simulink model "dcpController"  (R2016b)
settings: Solver=ode5  StartTime=0.0  StopTime=inf  FixedStep=0.001  RelTol=1e-3  EnableMultiTasking=on
undefined symbols (not defined in the file): robot, Standard_Devices, UDP_Protocol
libraries: dcpctrl x15, simulink x7, kukaslxctrl x1, sldrtlib x1
settings Model: SimulationMode=external  Creator=julianleland  LastModifiedBy=julianleland
settings OptimizationCC: LifeSpan=inf
settings DebuggingCC: SFUnexpectedBacktrackingDiag=warning  SFNoUnconditionalDefaultTransitionDiag=warning  SFExecutionAtInitializationDiag=none
settings HardwareCC: ProdBitPerLong=64  ProdHWDeviceType=Intel->x86-64 (Mac OS X)  TargetBitPerLong=64  TargetBitPerPointer=64  TargetIntDivRoundTo=Zero  TargetEndianess=LittleEndian  TargetWordSize=64  TargetHWDeviceType=Intel->x86-64
settings RTWCC: SystemTargetFile=sldrt.tlc  TemplateMakefile=sldrt.tmf  Description=Simulink Desktop Real-Time  RTWCompilerOptimization=on
settings CodeAppCC: MaxIdLength=95
settings SimulinkDesktopRealTimeCC: TargetPreCompLibLocation=/Applications/MATLAB_R2016b.app/toolbox/sldrt/lib/maci64  TargetLangStandard=C89/C90 (ANSI)  SupportVariableSizeSignals=off
settings ConfigComp: CovMetricSettings=dw  CovHtmlReporting=on  CovSaveCumulativeToWorkspaceVar=on  CovSaveSingleToWorkspaceVar=on  CovExternalEMLEnable=off

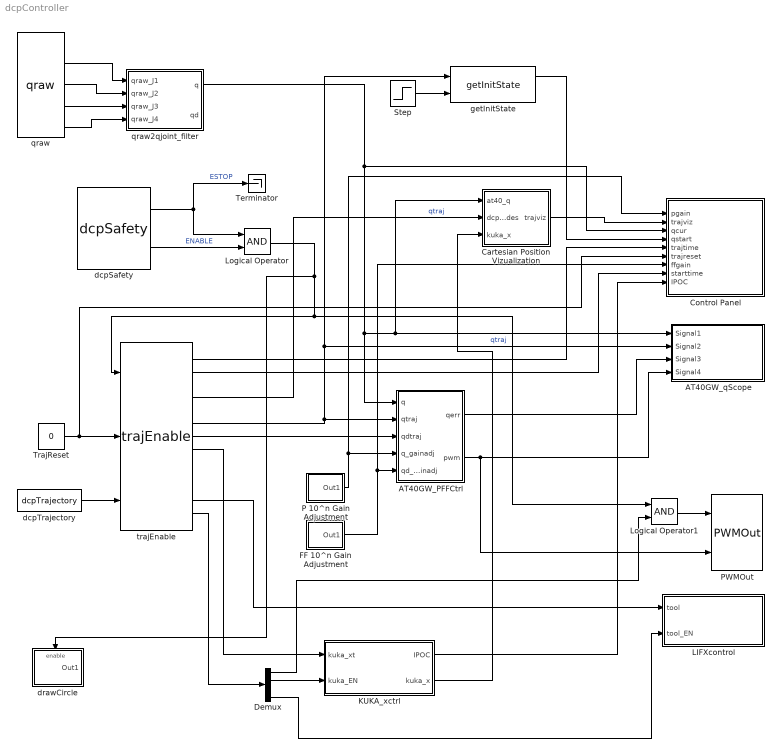
== system dcpController ==
  AT40GW_PFFCtrl : Subsystem
  AT40GW_qScope : Subsystem  AncestorBlock=dcpctrl/AT40GW_qScope
  Cartesian Position Vizualization : Subsystem
  Control Panel : Subsystem
  Demux : Demux
  FF 10^n Gain Adjustment : Subsystem
  KUKA_xctrl : Subsystem
  LIFXcontrol : Subsystem
  Logical Operator : Logic  AllPortsSameDT=off  OutDataTypeStr=boolean
  Logical Operator1 : Logic  AllPortsSameDT=off  OutDataTypeStr=boolean
  P 10^n Gain Adjustment : Subsystem
  PWMOut : dcpctrl/PWMOut
  Step : Step  Time=0  SampleTime=0
  Terminator : Terminator
  TrajReset : Constant  Value=0
  dcpSafety : dcpctrl/dcpSafety
  dcpTrajectory : dcpctrl/dcpTrajectory
  drawCircle : Subsystem
  getInitState : dcpctrl/getInitState
  qraw : dcpctrl/qraw
  qraw2qjoint_filter : Subsystem
  trajEnable : dcpctrl/trajEnable
      link override "Stoppable Time/Trajectory Time ": Gain=0
  wires:
  trajEnable/6 -> getInitState/1, AT40GW_qScope/2(Signal2), AT40GW_PFFCtrl/2(qtraj)  "qtraj"
  AT40GW_PFFCtrl/2(pwm) -> PWMOut/2, AT40GW_qScope/4(Signal4)
  AT40GW_PFFCtrl/1(qerr) -> AT40GW_qScope/3(Signal3)
  P 10^n Gain Adjustment/1(Out1) -> Control Panel/1(pgain), AT40GW_PFFCtrl/4("q_gainadj ")
  Logical Operator/1 -> drawCircle/Enable, Logical Operator1/1, trajEnable/1
  dcpSafety/1 -> Logical Operator/1, Terminator/1  "ESTOP"
  dcpSafety/2 -> Logical Operator/2  "ENABLE"
  TrajReset/1 -> Control Panel/6(trajreset), trajEnable/2
  getInitState/1 -> Control Panel/4(qstart)
  Step/1 -> getInitState/2
  trajEnable/1 -> Control Panel/5(trajtime)
  qraw2qjoint_filter/1(q) -> Control Panel/3(qcur), AT40GW_PFFCtrl/1(q), Cartesian Position Vizualization/1(at40_q), AT40GW_qScope/1(Signal1)
  FF 10^n Gain Adjustment/1(Out1) -> Control Panel/7(ffgain), AT40GW_PFFCtrl/5(qd_gainadj)
  trajEnable/7 -> AT40GW_PFFCtrl/3(qdtraj)
  trajEnable/12 -> LIFXcontrol/1(tool)
  dcpTrajectory/1 -> trajEnable/3
  trajEnable/2 -> Control Panel/8(starttime)
  qraw/2 -> qraw2qjoint_filter/1(qraw_J1)
  qraw/3 -> qraw2qjoint_filter/2(qraw_J2)
  qraw/4 -> qraw2qjoint_filter/3(qraw_J3)
  qraw/5 -> qraw2qjoint_filter/4(qraw_J4)
  Cartesian Position Vizualization/1(trajviz) -> Control Panel/2(trajviz)
  KUKA_xctrl/1(IPOC) -> Control Panel/9(IPOC)
  trajEnable/8 -> KUKA_xctrl/1("kuka_xt   ")
  Demux/2 -> KUKA_xctrl/2(kuka_EN)
  trajEnable/13 -> Demux/1
  Demux/4 -> LIFXcontrol/2(tool_EN)
  Logical Operator1/1 -> PWMOut/1
  Demux/1 -> Logical Operator1/2
  KUKA_xctrl/2(kuka_x) -> Cartesian Position Vizualization/3(kuka_x)
  trajEnable/4 -> Cartesian Position Vizualization/2(dcp_xdes)  "qtraj"

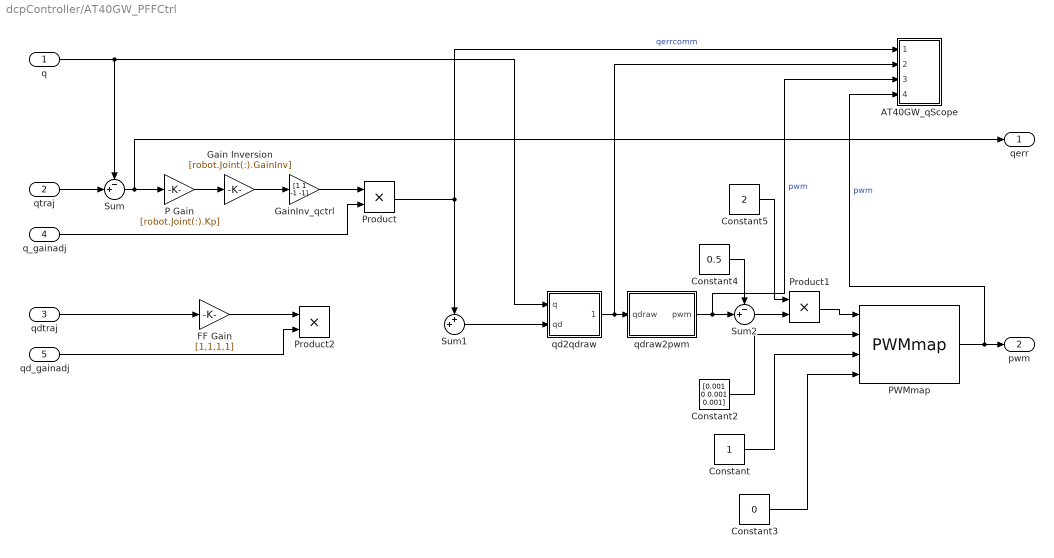
== system dcpController/AT40GW_PFFCtrl ==
  q : Inport
  qtraj : Inport  Port=2
  qdtraj : Inport  Port=3
  "q_gainadj " : Inport  Port=4
  qd_gainadj : Inport  Port=5
  AT40GW_qScope : Subsystem
  Constant : Constant
  Constant2 : Constant  Value=[0.001 0 0.001 0.001]
  Constant3 : Constant  Value=0
  Constant4 : Constant  Value=0.5
  Constant5 : Constant  Value=2
  FF Gain : Gain  Gain=[1,1,1,1]
  Gain Inversion : Gain  Gain=[robot.Joint(:).GainInv]
  GainInv_qctrl : Gain  Gain=[1 1 -1 -1]
  P Gain : Gain  Gain=[robot.Joint(:).Kp]
  PWMmap : dcpctrl/PWMmap
  Product : Product
  Product1 : Product
  Product2 : Product
  Sum : Sum  Inputs=-+|
  Sum1 : Sum  Inputs=++|
  Sum2 : Sum  Inputs=-+|
  qd2qdraw : Subsystem
  qdraw2pwm : Subsystem
  qerr : Outport
  pwm : Outport  Port=2
  wires:
  qtraj/1 -> Sum/2
  Sum/1 -> P Gain/1, qerr/1
  P Gain/1 -> Gain Inversion/1
  "q_gainadj "/1 -> Product/2
  Constant/1 -> PWMmap/3
  Constant3/1 -> PWMmap/4
  Constant2/1 -> PWMmap/2
  Gain Inversion/1 -> GainInv_qctrl/1
  Sum1/1 -> qd2qdraw/2(qd)
  q/1 -> qd2qdraw/1(q), Sum/1
  qd2qdraw/1(qdraw) -> AT40GW_qScope/2(Signal2), qdraw2pwm/1(qdraw)
  GainInv_qctrl/1 -> Product/1
  qdraw2pwm/1(pwm) -> AT40GW_qScope/3(Signal3), Sum2/2  "pwm"
  Constant4/1 -> Sum2/1
  Sum2/1 -> Product1/2
  Product1/1 -> PWMmap/1
  Constant5/1 -> Product1/1
  qd_gainadj/1 -> Product2/2
  qdtraj/1 -> FF Gain/1
  FF Gain/1 -> Product2/1
  PWMmap/1 -> AT40GW_qScope/4(Signal4), pwm/1  "pwm"
  Product/1 -> Sum1/1, AT40GW_qScope/1(Signal1)  "qerrcomm"

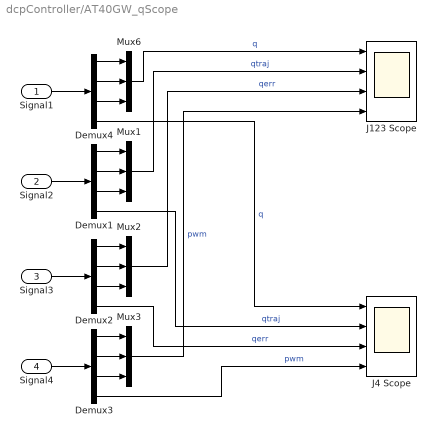
== system dcpController/AT40GW_qScope ==
  Signal1 : Inport
  Signal2 : Inport  Port=2
  Signal3 : Inport  Port=3
  Signal4 : Inport  Port=4
  Demux{1..4} (4 alike) : Demux
  J123 Scope : Scope  NumInputPorts=4
  J4 Scope : Scope  NumInputPorts=4
  Mux{1..3,6} (4 alike) : Mux  Inputs=3
  wires:
  Demux4/1 -> Mux6/1
  Mux3/1 -> J123 Scope/4  "pwm"
  Demux2/4 -> J4 Scope/3  "qerr"
  Demux1/4 -> J4 Scope/2  "qtraj"
  Mux6/1 -> J123 Scope/1  "q"
  Signal1/1 -> Demux4/1
  Demux4/2 -> Mux6/2
  Demux4/3 -> Mux6/3
  Demux1/1 -> Mux1/1
  Signal2/1 -> Demux1/1
  Demux1/2 -> Mux1/2
  Demux1/3 -> Mux1/3
  Demux2/1 -> Mux2/1
  Signal3/1 -> Demux2/1
  Demux2/2 -> Mux2/2
  Demux2/3 -> Mux2/3
  Demux3/1 -> Mux3/1
  Signal4/1 -> Demux3/1
  Demux3/2 -> Mux3/2
  Demux3/3 -> Mux3/3
  Mux1/1 -> J123 Scope/2  "qtraj"
  Mux2/1 -> J123 Scope/3  "qerr"
  Demux4/4 -> J4 Scope/1  "q"
  Demux3/4 -> J4 Scope/4  "pwm"

== system dcpController/Cartesian Position Vizualization ==
  at40_q : Inport
  dcp_xdes : Inport  Port=2
  kuka_x : Inport  Port=3
  Mux : Mux  Inputs=2
  Sum : Sum
  fkine_at40gw : MATLAB Function  TreatAsAtomicUnit=on
  trajviz : Outport
  wires:
  at40_q/1 -> fkine_at40gw/1(q)
  fkine_at40gw/1(x) -> Sum/2
  Mux/1 -> trajviz/1
  Sum/1 -> Mux/1
  kuka_x/1 -> Sum/1
  dcp_xdes/1 -> Mux/2

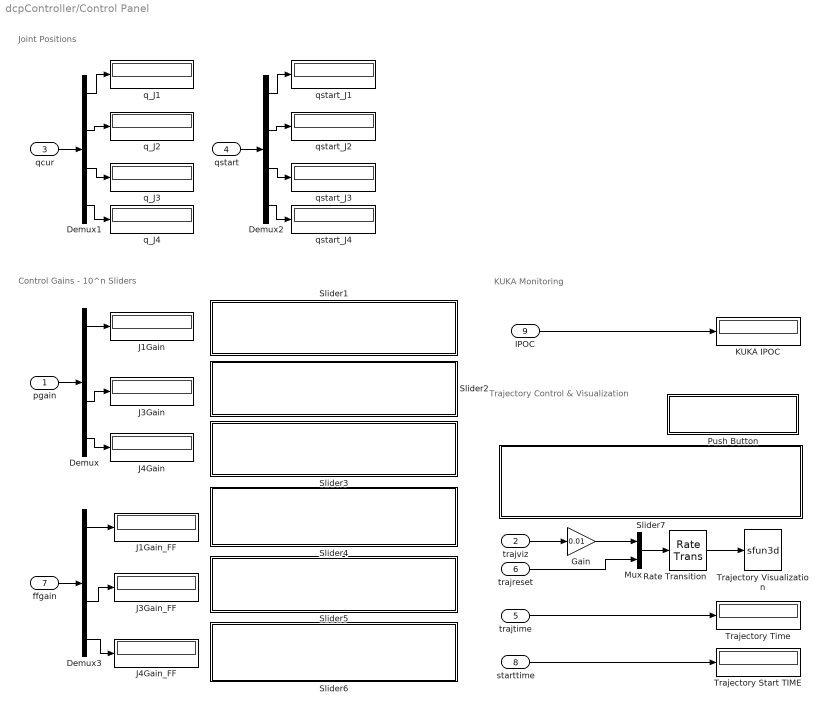
== system dcpController/Control Panel ==
  note: KUKA Monitoring
  note: Joint Positions
  note: Trajectory Control & Visualization
  note: Control Gains - 10^n Sliders
  pgain : Inport
  trajviz : Inport  Port=2
  qcur : Inport  Port=3
  qstart : Inport  Port=4
  trajtime : Inport  Port=5
  trajreset : Inport  Port=6
  ffgain : Inport  Port=7
  starttime : Inport  Port=8
  IPOC : Inport  Port=9
  Demux{,1..3} (4 alike) : Demux
  Gain : Gain  Gain=0.01
  J1Gain : Display
  J1Gain_FF : Display
  J3Gain : Display
  J3Gain_FF : Display
  J4Gain : Display
  J4Gain_FF : Display
  KUKA IPOC : Display
  Mux : Mux  Inputs=2
  Push Button : Subsystem  DialogController=hmiCreateDDGDialog  IsWebBlock=on  mask(MWDashboardBlock){webBlockId=d14440dc-dcfb-4a22-9820-9883405fda4f, webBlockType=pushbutton, ShowInLibBrwoser=on, ShowInitialText=on, HMISrcModelName=dcpController}
      mask prompts: webBlockId "WebBlock Id"; webBlockType "WebBlock Type"; HMISrcModelName "Source Model"
      mask Help: helpview([docroot '/mapfiles/simulink.map'], 'hmi_push_button')
      mask Display:
      | model = bdroot(gcb);
      | if strcmp(get_param(model,'BlockDiagramType'), 'library')
      |     image([(matlabroot) '/toolbox/simulink/hmi/icons/PushButton.png']);
      | end
  Rate Transition : RateTransition
  Slider1 : Subsystem  DialogController=hmiCreateDDGDialog  IsWebBlock=on  mask(MWDashboardBlock){webBlockId=1b4d9833-0382-4353-be8c-f20f38eb9aab, webBlockType=slider, ShowInLibBrowser=on, ShowInitialText=on, HMISrcModelName=dcpController}
      mask prompts: webBlockId "WebBlock Id"; webBlockType "WebBlock Type"; HMISrcModelName "Source Model"
      mask Help: helpview([docroot '/mapfiles/simulink.map'], 'hmi_slider')
      mask Display:
      | if strcmp(get_param(bdroot(gcb),'BlockDiagramType'), 'library')
      |     image([(matlabroot) '/toolbox/simulink/hmi/icons/Slider.png']);
      | end
  Slider2 : Subsystem  DialogController=hmiCreateDDGDialog  IsWebBlock=on  mask(MWDashboardBlock){webBlockId=cbf9babb-b489-42eb-b20a-0d2a912eb983, webBlockType=slider, ShowInLibBrowser=on, ShowInitialText=on, HMISrcModelName=dcpController}
      mask prompts: webBlockId "WebBlock Id"; webBlockType "WebBlock Type"; HMISrcModelName "Source Model"
      mask Help: helpview([docroot '/mapfiles/simulink.map'], 'hmi_slider')
      mask Display:
      | if strcmp(get_param(bdroot(gcb),'BlockDiagramType'), 'library')
      |     image([(matlabroot) '/toolbox/simulink/hmi/icons/Slider.png']);
      | end
  Slider3 : Subsystem  DialogController=hmiCreateDDGDialog  IsWebBlock=on  mask(MWDashboardBlock){webBlockId=af3345d3-46b3-4b00-a2f8-3f6dd7fd4884, webBlockType=slider, ShowInLibBrowser=on, ShowInitialText=on, HMISrcModelName=dcpController}
      mask prompts: webBlockId "WebBlock Id"; webBlockType "WebBlock Type"; HMISrcModelName "Source Model"
      mask Help: helpview([docroot '/mapfiles/simulink.map'], 'hmi_slider')
      mask Display:
      | if strcmp(get_param(bdroot(gcb),'BlockDiagramType'), 'library')
      |     image([(matlabroot) '/toolbox/simulink/hmi/icons/Slider.png']);
      | end
  Slider4 : Subsystem  DialogController=hmiCreateDDGDialog  IsWebBlock=on  mask(MWDashboardBlock){webBlockId=c89750c1-d32c-4c6a-899a-daca88898995, webBlockType=slider, ShowInLibBrowser=on, ShowInitialText=on, HMISrcModelName=dcpController}
      mask prompts: webBlockId "WebBlock Id"; webBlockType "WebBlock Type"; HMISrcModelName "Source Model"
      mask Help: helpview([docroot '/mapfiles/simulink.map'], 'hmi_slider')
      mask Display:
      | if strcmp(get_param(bdroot(gcb),'BlockDiagramType'), 'library')
      |     image([(matlabroot) '/toolbox/simulink/hmi/icons/Slider.png']);
      | end
  Slider5 : Subsystem  DialogController=hmiCreateDDGDialog  IsWebBlock=on  mask(MWDashboardBlock){webBlockId=a8dd70f1-7c39-409c-bbaa-299b93baa409, webBlockType=slider, ShowInLibBrowser=on, ShowInitialText=on, HMISrcModelName=dcpController}
      mask prompts: webBlockId "WebBlock Id"; webBlockType "WebBlock Type"; HMISrcModelName "Source Model"
      mask Help: helpview([docroot '/mapfiles/simulink.map'], 'hmi_slider')
      mask Display:
      | if strcmp(get_param(bdroot(gcb),'BlockDiagramType'), 'library')
      |     image([(matlabroot) '/toolbox/simulink/hmi/icons/Slider.png']);
      | end
  Slider6 : Subsystem  DialogController=hmiCreateDDGDialog  IsWebBlock=on  mask(MWDashboardBlock){webBlockId=99b5f6f1-a2e8-44e0-a565-9b4153c34515, webBlockType=slider, ShowInLibBrowser=on, ShowInitialText=on, HMISrcModelName=dcpController}
      mask prompts: webBlockId "WebBlock Id"; webBlockType "WebBlock Type"; HMISrcModelName "Source Model"
      mask Help: helpview([docroot '/mapfiles/simulink.map'], 'hmi_slider')
      mask Display:
      | if strcmp(get_param(bdroot(gcb),'BlockDiagramType'), 'library')
      |     image([(matlabroot) '/toolbox/simulink/hmi/icons/Slider.png']);
      | end
  Slider7 : Subsystem  DialogController=hmiCreateDDGDialog  IsWebBlock=on  mask(MWDashboardBlock){webBlockId=8192e4e1-ec01-457d-8e28-0b86459142e6, webBlockType=slider, ShowInLibBrowser=on, ShowInitialText=on, HMISrcModelName=dcpController}
      mask prompts: webBlockId "WebBlock Id"; webBlockType "WebBlock Type"; HMISrcModelName "Source Model"
      mask Help: helpview([docroot '/mapfiles/simulink.map'], 'hmi_slider')
      mask Display:
      | if strcmp(get_param(bdroot(gcb),'BlockDiagramType'), 'library')
      |     image([(matlabroot) '/toolbox/simulink/hmi/icons/Slider.png']);
      | end
  Trajectory Visualization : S-Function  LoadFcn=if exist('sfun3d','file'), sfun3d([],[],[],'LoadBlock'); end  FunctionName=sfun3d  Parameters=ax,T,np,cp,gd,ls,mk  SFunctionDeploymentMode=off  EnableBusSupport=off  mask(3D Graph){np=2, ax=[30 80 -20 20 -10 30], cp=[80 10 20], gd=on, ls=-, mk=., T=0.1}
      mask prompts: np "Number of point (lines)"; ax "[xmin xmax  ymin ymax zmin zmax]"; cp "Camera position (use [0 0 1] for 2D XY view)"; gd "Grid (on|off)"; ls "LineStyle"; mk "Marker"; T "Sampling Time"
      mask help:
      | This block plots the position of several points in the XYZ space. The input contains the coordinates of all the points (x1,y1,z1,x2,y2,z2,...).
      | The number of points (lines), the XYZ ranges, camera position, grid, linestyle, marker and sampling time, can be set as mask parameters.
      settings: CopyFcn=if exist('sfun3d','file'), sfun3d([],[],[],'CopyBlock'); end  DeleteFcn=if exist('sfun3d','file'), sfun3d([],[],[],'DeleteBlock'); end  NameChangeFcn=if exist('sfun3d','file'), sfun3d([],[],[],'NameChange'); end
      mask Help:
      | This block plots the position of several points in the XYZ space. The input contains the coordinates of all the points (x1,y1,z1,x2,y2,z2,...).
      | The number of points (lines), the XYZ ranges, camera position, grid, linestyle, marker and sampling time, can be set as mask parameters.
      mask TypeOptions ls: - | -- | : | -. | none
      mask TypeOptions mk: none | . | + | o | * | x | square | diamond | v | ^ | > | < | pentagram | hexagram
      mask Display: plot([.05 .95 .95 .05 .05],[.45 .45 .95 .95 .45], 0.5+cos(0:0.1:2*pi)*0.3,0.7+sin(0:0.1:2*pi)*0.2)
  Trajectory Start TIME : Display
  Trajectory Time : Display
  q_J{1..4} (4 alike) : Display
  qstart_J{1..4} (4 alike) : Display
  wires:
  pgain/1 -> Demux/1
  Demux/4 -> J4Gain/1
  Demux/1 -> J1Gain/1
  Demux/3 -> J3Gain/1
  qcur/1 -> Demux1/1
  Demux1/4 -> q_J4/1
  Demux1/1 -> q_J1/1
  Demux1/3 -> q_J3/1
  Demux1/2 -> q_J2/1
  qstart/1 -> Demux2/1
  Demux2/4 -> qstart_J4/1
  Demux2/1 -> qstart_J1/1
  Demux2/3 -> qstart_J3/1
  Demux2/2 -> qstart_J2/1
  trajtime/1 -> Trajectory Time/1
  ffgain/1 -> Demux3/1
  Demux3/4 -> J4Gain_FF/1
  Demux3/1 -> J1Gain_FF/1
  Demux3/3 -> J3Gain_FF/1
  trajviz/1 -> Gain/1
  Gain/1 -> Mux/1
  Mux/1 -> Rate Transition/1
  Rate Transition/1 -> Trajectory Visualization/1
  trajreset/1 -> Mux/2
  starttime/1 -> Trajectory Start TIME/1
  IPOC/1 -> KUKA IPOC/1

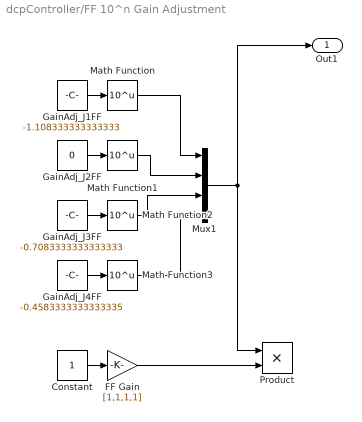
== system dcpController/FF 10^n Gain Adjustment ==
  Constant : Constant
  FF Gain : Gain  Gain=[1,1,1,1]
  GainAdj_J1FF : Constant  Value=-1.108333333333333
  GainAdj_J2FF : Constant  Value=0
  GainAdj_J3FF : Constant  Value=-0.7083333333333333
  GainAdj_J4FF : Constant  Value=-0.4583333333333335
  Math Function{,1..3} (4 alike) : Math  Operator=10^u  SaturateOnIntegerOverflow=on
  Mux1 : Mux
  Product : Product
  Out1 : Outport
  wires:
  Math Function1/1 -> Mux1/2
  Math Function/1 -> Mux1/1
  Mux1/1 -> Out1/1, Product/1
  Math Function3/1 -> Mux1/4
  Math Function2/1 -> Mux1/3
  GainAdj_J1FF/1 -> Math Function/1
  GainAdj_J2FF/1 -> Math Function1/1
  GainAdj_J3FF/1 -> Math Function2/1
  GainAdj_J4FF/1 -> Math Function3/1
  Constant/1 -> FF Gain/1
  FF Gain/1 -> Product/2

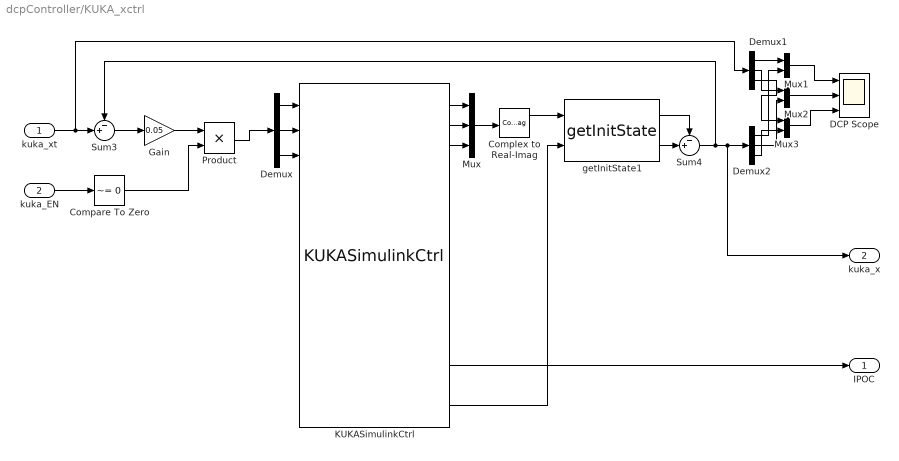
== system dcpController/KUKA_xctrl ==
  "kuka_xt   " : Inport
  kuka_EN : Inport  Port=2
  Compare To Zero : simulink/Logic and Bit Operations/Compare To Zero  relop=~=  OutDataTypeStr=boolean
  Complex to Real-Imag : ComplexToRealImag
  DCP Scope : Scope  NumInputPorts=3
  Demux : Demux  Outputs=3
  Demux1 : Demux  Outputs=3
  Demux2 : Demux  Outputs=3
  Gain : Gain  Gain=0.05
  KUKASimulinkCtrl : kukaslxctrl/KUKASimulinkCtrl
  Mux : Mux  Inputs=3
  Mux1 : Mux  Inputs=2
  Mux2 : Mux  Inputs=2
  Mux3 : Mux  Inputs=2
  Product : Product
  Sum3 : Sum  Inputs=-+|
  Sum4 : Sum  Inputs=-+|
  getInitState1 : dcpctrl/getInitState
  IPOC : Outport
  kuka_x : Outport  Port=2
  wires:
  KUKASimulinkCtrl/16 -> getInitState1/2
  KUKASimulinkCtrl/2 -> Mux/2
  Sum4/1 -> kuka_x/1, Demux2/1, Sum3/1
  KUKASimulinkCtrl/14 -> IPOC/1
  KUKASimulinkCtrl/1 -> Mux/1
  Complex to Real-Imag/1 -> getInitState1/1
  KUKASimulinkCtrl/3 -> Mux/3
  Demux/2 -> KUKASimulinkCtrl/2
  Demux/3 -> KUKASimulinkCtrl/3
  Mux/1 -> Complex to Real-Imag/1
  getInitState1/1 -> Sum4/1
  getInitState1/2 -> Sum4/2
  Demux/1 -> KUKASimulinkCtrl/1
  Demux1/1 -> Mux1/1
  Mux1/1 -> DCP Scope/1
  Demux2/1 -> Mux1/2
  Mux2/1 -> DCP Scope/2
  Demux1/2 -> Mux2/1
  Mux3/1 -> DCP Scope/3
  Demux2/3 -> Mux3/2
  Demux2/2 -> Mux2/2
  Demux1/3 -> Mux3/1
  "kuka_xt   "/1 -> Sum3/2, Demux1/1
  Sum3/1 -> Gain/1
  kuka_EN/1 -> Compare To Zero/1
  Gain/1 -> Product/1
  Product/1 -> Demux/1
  Compare To Zero/1 -> Product/2

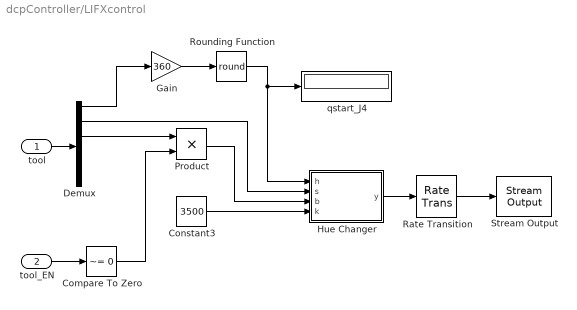
== system dcpController/LIFXcontrol ==
  tool : Inport
  tool_EN : Inport  Port=2
  Compare To Zero : simulink/Logic and Bit Operations/Compare To Zero  relop=~=  OutDataTypeStr=boolean
  Constant3 : Constant  Value=3500  OutMin=[2500]  OutMax=[9000]  OutDataTypeStr=double
  Demux : Demux  Outputs=6
  Gain : Gain  Gain=360
  Hue Changer : MATLAB Function  TreatAsAtomicUnit=on
  Product : Product
  Rate Transition : RateTransition
  Rounding Function : Rounding  Operator=round
  Stream Output : sldrtlib/Stream Output  SampleTime=.1  MaxMissedTicks=10  ShowMissedTicks=off  YieldWhenWaiting=on  DrvName=Standard_Devices/UDP_Protocol  DrvAddress=54359  DrvOptions=[174338150 56700]  PortSizes=49  FormatString=repmat('%c',1,49)  ShowReady=off  ShowError=off  InitialValue=[]  FinalValue=[]
      settings: AttributesFormatString=Standard Devices\nUDP Protocol [D457h]
  qstart_J4 : Display
  wires:
  Hue Changer/1(y) -> Rate Transition/1
  Demux/2 -> Hue Changer/2(s)
  Constant3/1 -> Hue Changer/4(k)
  Rounding Function/1 -> Hue Changer/1(h), qstart_J4/1
  tool/1 -> Demux/1
  Rate Transition/1 -> Stream Output/1
  Demux/1 -> Gain/1
  Gain/1 -> Rounding Function/1
  tool_EN/1 -> Compare To Zero/1
  Compare To Zero/1 -> Product/2
  Demux/3 -> Product/1
  Product/1 -> Hue Changer/3(b)

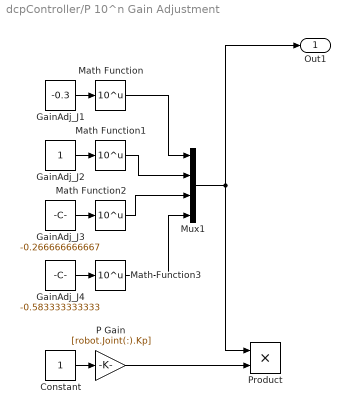
== system dcpController/P 10^n Gain Adjustment ==
  Constant : Constant
  GainAdj_J1 : Constant  Value=-0.3
  GainAdj_J2 : Constant
  GainAdj_J3 : Constant  Value=-0.266666666667
  GainAdj_J4 : Constant  Value=-0.583333333333
  Math Function{,1..3} (4 alike) : Math  Operator=10^u  SaturateOnIntegerOverflow=on
  Mux1 : Mux
  P Gain : Gain  Gain=[robot.Joint(:).Kp]
  Product : Product
  Out1 : Outport
  wires:
  Math Function1/1 -> Mux1/2
  Math Function/1 -> Mux1/1
  Mux1/1 -> Out1/1, Product/1
  Math Function3/1 -> Mux1/4
  Math Function2/1 -> Mux1/3
  GainAdj_J1/1 -> Math Function/1
  GainAdj_J2/1 -> Math Function1/1
  GainAdj_J3/1 -> Math Function2/1
  GainAdj_J4/1 -> Math Function3/1
  Constant/1 -> P Gain/1
  P Gain/1 -> Product/2

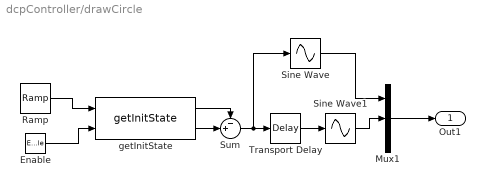
== system dcpController/drawCircle ==
  Enable : EnablePort  ShowOutputPort=on
  Mux1 : Mux  Inputs=3
  Ramp : simulink/Sources/Ramp  slope=1  start=0  X0=0
  Sine Wave : Sin  TimeSource=Use external signal  Amplitude=200  Frequency=0.5  SampleTime=0
  Sine Wave1 : Sin  TimeSource=Use external signal  Amplitude=200  Frequency=0.5  SampleTime=0
  Sum : Sum  Inputs=-+|
  Transport Delay : TransportDelay  DelayTime=3
  getInitState : dcpctrl/getInitState
  Out1 : Outport
  wires:
  Sine Wave/1 -> Mux1/1
  Sine Wave1/1 -> Mux1/2
  Mux1/1 -> Out1/1
  Enable/1 -> getInitState/2
  Ramp/1 -> getInitState/1
  getInitState/2 -> Sum/2
  getInitState/1 -> Sum/1
  Sum/1 -> Transport Delay/1, Sine Wave/1
  Transport Delay/1 -> Sine Wave1/1

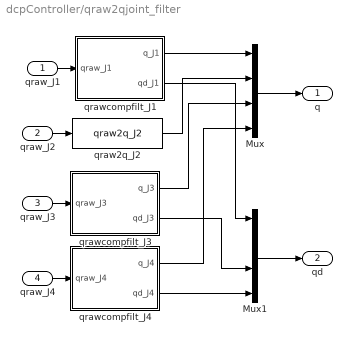
== system dcpController/qraw2qjoint_filter ==
  qraw_J1 : Inport
  qraw_J2 : Inport  Port=2
  qraw_J3 : Inport  Port=3
  qraw_J4 : Inport  Port=4
  Mux : Mux
  Mux1 : Mux
  qraw2q_J2 : dcpctrl/qraw2q_J2
  qrawcompfilt_J1 : Subsystem
  qrawcompfilt_J3 : Subsystem
  qrawcompfilt_J4 : Subsystem
  q : Outport
  qd : Outport  Port=2
  wires:
  qraw_J2/1 -> qraw2q_J2/1
  qraw_J1/1 -> qrawcompfilt_J1/1(qraw_J1)
  qraw_J4/1 -> qrawcompfilt_J4/1(qraw_J4)
  qraw_J3/1 -> qrawcompfilt_J3/1(qraw_J3)
  qrawcompfilt_J4/2(qd_J4) -> Mux1/4
  qrawcompfilt_J3/2(qd_J3) -> Mux1/3
  qrawcompfilt_J1/2(qd_J1) -> Mux1/1
  qrawcompfilt_J1/1(q_J1) -> Mux/1
  qraw2q_J2/1 -> Mux/2
  qrawcompfilt_J3/1(q_J3) -> Mux/3
  qrawcompfilt_J4/1(q_J4) -> Mux/4
  Mux1/1 -> qd/1
  Mux/1 -> q/1

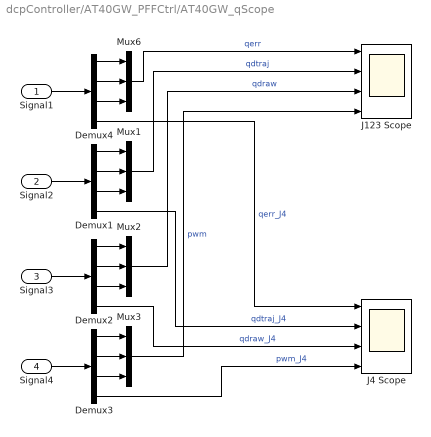
== system dcpController/AT40GW_PFFCtrl/AT40GW_qScope ==
  Signal1 : Inport
  Signal2 : Inport  Port=2
  Signal3 : Inport  Port=3
  Signal4 : Inport  Port=4
  Demux{1..4} (4 alike) : Demux
  J123 Scope : Scope  NumInputPorts=4
  J4 Scope : Scope  NumInputPorts=4
  Mux{1..3,6} (4 alike) : Mux  Inputs=3
  wires:
  Mux3/1 -> J123 Scope/4  "pwm"
  Demux2/4 -> J4 Scope/3  "qdraw_J4"
  Demux1/4 -> J4 Scope/2  "qdtraj_J4"
  Mux6/1 -> J123 Scope/1  "qerr"
  Signal1/1 -> Demux4/1
  Demux4/2 -> Mux6/2
  Demux4/3 -> Mux6/3
  Demux1/1 -> Mux1/1
  Signal2/1 -> Demux1/1
  Demux1/2 -> Mux1/2
  Demux1/3 -> Mux1/3
  Signal3/1 -> Demux2/1
  Demux2/2 -> Mux2/2
  Demux2/3 -> Mux2/3
  Demux3/1 -> Mux3/1
  Signal4/1 -> Demux3/1
  Demux3/2 -> Mux3/2
  Demux3/3 -> Mux3/3
  Mux1/1 -> J123 Scope/2  "qdtraj"
  Mux2/1 -> J123 Scope/3  "qdraw"
  Demux4/4 -> J4 Scope/1  "qerr_J4"
  Demux3/4 -> J4 Scope/4  "pwm_J4"
  Demux2/1 -> Mux2/1
  Demux4/1 -> Mux6/1

== system dcpController/AT40GW_PFFCtrl/qd2qdraw ==
  q : Inport
  qd : Inport  Port=2
  dj2drfcn : MATLAB Function  TreatAsAtomicUnit=on
  qdraw : Outport
  wires:
  qd/1 -> dj2drfcn/2(qd)
  dj2drfcn/1(qdraw) -> qdraw/1
  q/1 -> dj2drfcn/1(q)

== system dcpController/AT40GW_PFFCtrl/qdraw2pwm ==
  qdraw : Inport
  Demux : Demux
  Mux : Mux
  qdraw2pwm_J1 : Subsystem
  qdraw2pwm_J2 : Subsystem
  qdraw2pwm_J3 : Subsystem
  qdraw2pwm_J4 : Subsystem
  pwm : Outport
  wires:
  qdraw/1 -> Demux/1
  Demux/1 -> qdraw2pwm_J1/1(qdraw_J1)
  Demux/3 -> qdraw2pwm_J3/1(qdraw_J3)
  Demux/2 -> qdraw2pwm_J2/1(qdraw_J2)
  Demux/4 -> qdraw2pwm_J4/1(qdraw_J4)
  qdraw2pwm_J4/1(pwm_J4) -> Mux/4
  qdraw2pwm_J3/1(pwm_J3) -> Mux/3
  Mux/1 -> pwm/1
  qdraw2pwm_J2/1(pwm_J2) -> Mux/2
  qdraw2pwm_J1/1(pwm_J1) -> Mux/1

== system dcpController/Control Panel/Push Button ==

== system dcpController/Control Panel/Slider1 ==

== system dcpController/Control Panel/Slider2 ==

== system dcpController/Control Panel/Slider3 ==

== system dcpController/Control Panel/Slider4 ==

== system dcpController/Control Panel/Slider5 ==

== system dcpController/Control Panel/Slider6 ==

== system dcpController/Control Panel/Slider7 ==

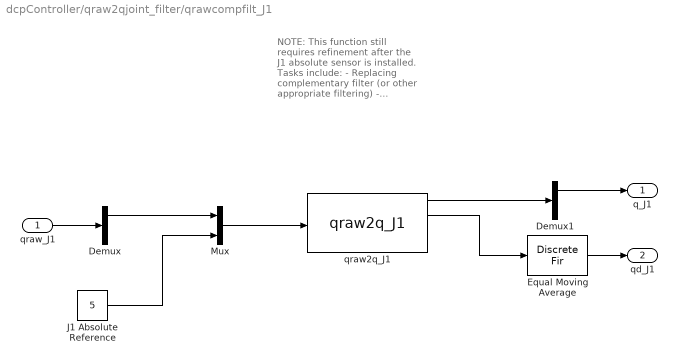
== system dcpController/qraw2qjoint_filter/qrawcompfilt_J1 ==
  note: NOTE: This function still requires refinement after the J1 absolute sensor is installed. Tasks include:
      | - Replacing complementary filter (or other appropriate filtering)
      | - Re-enabling J1 absolute input (removing J1 Absolute Reference block)
  qraw_J1 : Inport
  Demux : Demux  Outputs=2
  Demux1 : Demux  Outputs=2
  Equal Moving Average : DiscreteFir  Coefficients=[0.1 0.1 0.1 0.1 0.1 0.1 0.1 0.1 0.1 0.1]  InputProcessing=Columns as channels (frame based)
  J1 Absolute Reference : Constant  Value=5
  Mux : Mux  Inputs=2
  qraw2q_J1 : dcpctrl/qraw2q_J1
  q_J1 : Outport
  qd_J1 : Outport  Port=2
  wires:
  qraw2q_J1/1 -> Demux1/1
  qraw2q_J1/2 -> Equal Moving Average/1
  Equal Moving Average/1 -> qd_J1/1
  Demux1/1 -> q_J1/1
  qraw_J1/1 -> Demux/1
  Demux/1 -> Mux/1
  Mux/1 -> qraw2q_J1/1
  J1 Absolute Reference/1 -> Mux/2

== system dcpController/qraw2qjoint_filter/qrawcompfilt_J3 ==
  qraw_J3 : Inport
  Complementary Filter : dcpctrl/complementaryFilter
  Demux1 : Demux  Outputs=2
  Equal Moving Average : DiscreteFir  Coefficients=[0.1 0.1 0.1 0.1 0.1 0.1 0.1 0.1 0.1 0.1]  InputProcessing=Columns as channels (frame based)
  Mux1 : Mux  Inputs=3
  compFiltTau_J4 : Constant  Value=0.036
  qraw2q_J3 : dcpctrl/qraw2q_J3
  q_J3 : Outport
  qd_J3 : Outport  Port=2
  wires:
  Complementary Filter/1 -> q_J3/1
  Equal Moving Average/1 -> qd_J3/1
  qraw_J3/1 -> qraw2q_J3/1
  Demux1/2 -> Complementary Filter/2, Mux1/1
  Demux1/1 -> Mux1/2
  qraw2q_J3/2 -> Complementary Filter/1, Equal Moving Average/1
  compFiltTau_J4/1 -> Complementary Filter/3
  qraw2q_J3/1 -> Demux1/1

== system dcpController/qraw2qjoint_filter/qrawcompfilt_J4 ==
  qraw_J4 : Inport
  Complementary Filter : dcpctrl/complementaryFilter
  Demux1 : Demux  Outputs=2
  Equal Moving Average : DiscreteFir  Coefficients=[0.1 0.1 0.1 0.1 0.1 0.1 0.1 0.1 0.1 0.1]  InputProcessing=Columns as channels (frame based)
  Mux1 : Mux  Inputs=3
  compFiltTau_J4 : Constant  Value=0.036
  qraw2q_J4 : dcpctrl/qraw2q_J4
  q_J4 : Outport
  qd_J4 : Outport  Port=2
  wires:
  qraw2q_J4/1 -> Demux1/1
  compFiltTau_J4/1 -> Complementary Filter/3
  qraw2q_J4/2 -> Equal Moving Average/1, Complementary Filter/1
  Demux1/1 -> Mux1/2
  Demux1/2 -> Mux1/1, Complementary Filter/2
  qraw_J4/1 -> qraw2q_J4/1
  Equal Moving Average/1 -> qd_J4/1
  Complementary Filter/1 -> Mux1/3, q_J4/1

== system dcpController/AT40GW_PFFCtrl/qdraw2pwm/qdraw2pwm_J1 ==
  qdraw_J1 : Inport
  Lookup Table Dynamic_J1 : simulink/Lookup Tables/Lookup Table Dynamic  LookUpMeth=Interpolation-Use End Values  OutDataType=fixdt('double')  OutScaling=[]  OutputDataTypeScalingMode=Specify via dialog  OutDataTypeStr=fixdt('double')  DoSatur=off
  pwm : FromWorkspace  VariableName=robot.J1qdr2PWMmap(:,1)'  SampleTime=0
  qdr : FromWorkspace  VariableName=robot.J1qdr2PWMmap(:,2)'  SampleTime=0
  pwm_J1 : Outport
  wires:
  Lookup Table Dynamic_J1/1 -> pwm_J1/1
  qdraw_J1/1 -> Lookup Table Dynamic_J1/1
  qdr/1 -> Lookup Table Dynamic_J1/2
  pwm/1 -> Lookup Table Dynamic_J1/3

== system dcpController/AT40GW_PFFCtrl/qdraw2pwm/qdraw2pwm_J2 ==
  qdraw_J2 : Inport
  Lookup Table Dynamic_J2 : simulink/Lookup Tables/Lookup Table Dynamic  LookUpMeth=Interpolation-Use End Values  OutDataType=fixdt('double')  OutScaling=[]  OutputDataTypeScalingMode=Specify via dialog  OutDataTypeStr=fixdt('double')  DoSatur=off
  pwm : FromWorkspace  VariableName=robot.J2qdr2PWMmap(:,1)'  SampleTime=0
  qdraw : FromWorkspace  VariableName=robot.J2qdr2PWMmap(:,2)'  SampleTime=0
  pwm_J2 : Outport
  wires:
  Lookup Table Dynamic_J2/1 -> pwm_J2/1
  qdraw_J2/1 -> Lookup Table Dynamic_J2/1
  qdraw/1 -> Lookup Table Dynamic_J2/2
  pwm/1 -> Lookup Table Dynamic_J2/3

== system dcpController/AT40GW_PFFCtrl/qdraw2pwm/qdraw2pwm_J3 ==
  qdraw_J3 : Inport
  Lookup Table DynamicJ3 : simulink/Lookup Tables/Lookup Table Dynamic  LookUpMeth=Interpolation-Use End Values  OutDataType=fixdt('double')  OutScaling=[]  OutputDataTypeScalingMode=Specify via dialog  OutDataTypeStr=fixdt('double')  DoSatur=off
  pwm : FromWorkspace  VariableName=robot.J3qdr2PWMmap(:,1)'  SampleTime=0
  qdraw : FromWorkspace  VariableName=robot.J3qdr2PWMmap(:,2)'  SampleTime=0
  pwm_J3 : Outport
  wires:
  Lookup Table DynamicJ3/1 -> pwm_J3/1
  qdraw_J3/1 -> Lookup Table DynamicJ3/1
  qdraw/1 -> Lookup Table DynamicJ3/2
  pwm/1 -> Lookup Table DynamicJ3/3

== system dcpController/AT40GW_PFFCtrl/qdraw2pwm/qdraw2pwm_J4 ==
  qdraw_J4 : Inport
  Lookup Table Dynamic_J4 : simulink/Lookup Tables/Lookup Table Dynamic  LookUpMeth=Interpolation-Use End Values  OutDataType=fixdt('double')  OutScaling=[]  OutputDataTypeScalingMode=Specify via dialog  OutDataTypeStr=fixdt('double')  DoSatur=off
  pwm : FromWorkspace  VariableName=robot.J4qdr2PWMmap(:,1)'  SampleTime=0
  qdraw : FromWorkspace  VariableName=robot.J4qdr2PWMmap(:,2)'  SampleTime=0
  pwm_J4 : Outport
  wires:
  Lookup Table Dynamic_J4/1 -> pwm_J4/1
  qdraw_J4/1 -> Lookup Table Dynamic_J4/1
  qdraw/1 -> Lookup Table Dynamic_J4/2
  pwm/1 -> Lookup Table Dynamic_J4/3

== matlab function dcpController/Cartesian Position Vizualization/fkine_at40gw ==
  data: q input; x output
function x = fcn(q)
%#codegen

x_temp = fkine_at40gw(q(1),q(2),q(3),q(4))*[1;0;0;0];
x = x_temp(2:4);

== matlab function dcpController/AT40GW_PFFCtrl/qd2qdraw/dj2drfcn ==
  data: q input; qdraw output; qd input
function qdraw = fcn(q,qd)
%#codegen

qdraw = dj2drfcn_at40gw(q(2),q(3))*qd;

== matlab function dcpController/LIFXcontrol/Hue Changer ==
  data: h input; y output size=[1,49]; s input; b input; k input
function y = fcn(h,s,b,k)
%#codegen
%%
dec_code = [49;0;0;52;0;0;0;0;0;0;0;0;0;0;0;0;0;0;0;0;0;0;0;0;0;0;0;0;0;0;0;0;102;0;0;0;0;85;85;255;255;255;255;191;218;0;0;0;0];
%%
%%HUE 
hue = h/360 * 65535; %hue conversion formula, from degrees scale to LIFX scale
hue = floor(hue);
hue_hex = dec2hex(hue);

if (length(hue_hex) == 1)
    hue_arr = ['0',hue_hex(1)];
    hue_arr = ['00',hue_arr(1:2)];

elseif (length(hue_hex) ==2)
    hue_arr = ['00',hue_hex(1:2)];  
    
elseif (length(hue_hex) == 3)
    hue_arr = ['0', hue_hex(1), hue_hex(2), hue_hex(3)];
    hue_arr = [hue_arr(1:2),hue_arr(3:4)];
    
else
    hue_arr = [hue_hex(1:2), hue_hex(3:4)];
        
end

hue_out = hex2dec(hue_arr(1:2));
hue_out2 = hex2dec(hue_arr(3:4));

dec_code(38) = hue_out2;
dec_code(39) = hue_out;

%%
%SATURATION
sat = s * 65535; %saturation conversion formula, from 0-1 to LIFX scale
sat = floor(sat);
sat_hex = dec2hex(sat);

if (length(sat_hex) == 1)
    sat_arr = ['0',sat_hex(1)];
    sat_arr = ['00',sat_arr(1:2)];

elseif (length(sat_hex) ==2)
    sat_arr = ['00',sat_hex(1:2)];  
    
elseif (length(sat_hex) == 3)
    sat_arr = ['0', sat_hex(1), sat_hex(2), sat_hex(3)];
    sat_arr = [sat_arr(1:2),sat_arr(3:4)];
    
else
    sat_arr = [sat_hex(1:2), sat_hex(3:4)];
        
end

sat_out = hex2dec(sat_arr(1:2));
sat_out2 = hex2dec(sat_arr(3:4));

dec_code(40) = sat_out2;
dec_code(41) = sat_out;

%%

%BRIGHTNESS
bright = b * 65535; %brightness conversion formula, from 0-1 to LIFX scale
bright = floor(bright);
bright_hex = dec2hex(bright);

if (length(bright_hex) == 1)
    bright_arr = ['0',bright_hex(1)];
    bright_arr = ['00',bright_arr(1:2)];

elseif (length(bright_hex) ==2)
    bright_arr = ['00',bright_hex(1:2)];  
    
elseif (length(bright_hex) == 3)
    bright_arr = ['0', bright_hex(1), bright_hex(2), bright_hex(3)];
    bright_arr = [bright_arr(1:2),bright_arr(3:4)];
    
else
    bright_arr = [bright_hex(1:2), bright_hex(3:4)];
end

bright_out = hex2dec(bright_arr(1:2));
bright_out2 = hex2dec(bright_arr(3:4));

dec_code(42) = bright_out2;
dec_code(43) = bright_out;

%%
%KELVIN
kelvin = k; %Kelvin conversion formula, from 0-1 to LIFX scale
kelvin = floor(kelvin);
kelvin_hex = dec2hex(kelvin);

if (length(kelvin_hex) == 1)
    kelvin_arr = ['0',kelvin_hex(1)];
    kelvin_arr = ['00',kelvin_arr(1:2)];

elseif (length(kelvin_hex) ==2)
    kelvin_arr = ['00',kelvin_hex(1:2)];  
    
elseif (length(kelvin_hex) == 3)
    kelvin_arr = ['0', kelvin_hex(1), kelvin_hex(2), kelvin_hex(3)];
    kelvin_arr = [kelvin_arr(1:2), kelvin_arr(3:4)];
    
else
    kelvin_arr = [kelvin_hex(1:2), kelvin_hex(3:4)];
end

kelvin_out = hex2dec(kelvin_arr(1:2));
kelvin_out2 = hex2dec(kelvin_arr(3:4));

dec_code(44) = kelvin_out2;
dec_code(45) = kelvin_out;

%%
%y_temp = char_out;
%y = y_temp(1:2);

y = uint8(dec_code');
